simulink model "ODWRobot_KinematicModel"  (R2019b)
settings: Solver=ode5  StartTime=0.0  StopTime=10  FixedStep=Ts  RelTol=1e-3
undefined symbols (not defined in the file or in its folder): b, k1, k2, phi_init, rw, x_init, y_init
libraries: simulink x1
settings Model: Creator=kerrm  LastModifiedBy=kerrm
settings DataIOCC: ReturnWorkspaceOutputs=off

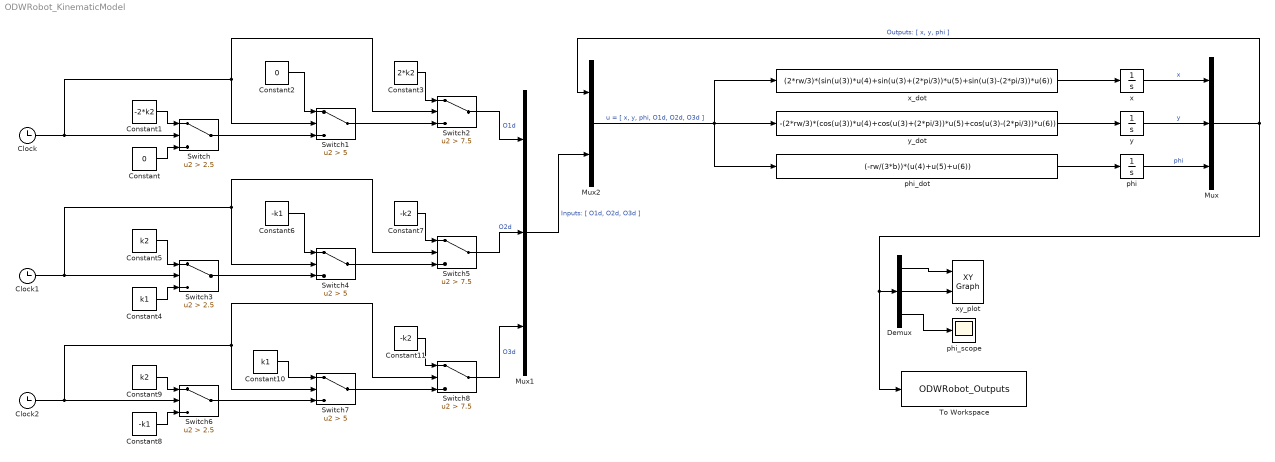
== system ODWRobot_KinematicModel ==
  Clock : Clock
  Clock1 : Clock
  Clock2 : Clock
  Constant : Constant  Value=0
  Constant1 : Constant  Value=-2*k2
  Constant10 : Constant  Value=k1
  Constant11 : Constant  Value=-k2
  Constant2 : Constant  Value=0
  Constant3 : Constant  Value=2*k2
  Constant4 : Constant  Value=k1
  Constant5 : Constant  Value=k2
  Constant6 : Constant  Value=-k1
  Constant7 : Constant  Value=-k2
  Constant8 : Constant  Value=-k1
  Constant9 : Constant  Value=k2
  Demux : Demux  Outputs=3
  Mux : Mux  Inputs=3
  Mux1 : Mux  Inputs=3
  Mux2 : Mux  Inputs=2
  Switch : Switch  Criteria=u2 > Threshold  Threshold=2.5
  Switch1 : Switch  Criteria=u2 > Threshold  Threshold=5
  Switch2 : Switch  Criteria=u2 > Threshold  Threshold=7.5
  Switch3 : Switch  Criteria=u2 > Threshold  Threshold=2.5
  Switch4 : Switch  Criteria=u2 > Threshold  Threshold=5
  Switch5 : Switch  Criteria=u2 > Threshold  Threshold=7.5
  Switch6 : Switch  Criteria=u2 > Threshold  Threshold=2.5
  Switch7 : Switch  Criteria=u2 > Threshold  Threshold=5
  Switch8 : Switch  Criteria=u2 > Threshold  Threshold=7.5
  To Workspace : ToWorkspace  VariableName=ODWRobot_Outputs  SampleTime=-1
      settings: Save2DSignal=2-D array (concatenate along first dimension)
  phi : Integrator  InitialCondition=phi_init
  phi_dot : Fcn  Expr=(-rw/(3*b))*(u(4)+u(5)+u(6))
  phi_scope : Scope
  x : Integrator  InitialCondition=x_init
  x_dot : Fcn  Expr=(2*rw/3)*(sin(u(3))*u(4)+sin(u(3)+(2*pi/3))*u(5)+sin(u(3)-(2*pi/3))*u(6))
  xy_plot : simulink/Sinks/XY Graph  xmin=-.1  xmax=1.1  ymin=-.1  ymax=1.1  st=-1
  y : Integrator  InitialCondition=y_init
  y_dot : Fcn  Expr=-(2*rw/3)*(cos(u(3))*u(4)+cos(u(3)+(2*pi/3))*u(5)+cos(u(3)-(2*pi/3))*u(6))
  wires:
  y/1 -> Mux/2  "y"
  phi/1 -> Mux/3  "phi"
  x/1 -> Mux/1  "x"
  Mux/1 -> To Workspace/1, Demux/1, Mux2/1  "Outputs: [ x, y, phi ]"
  Mux1/1 -> Mux2/2  "Inputs: [ O1d, O2d, O3d ]"
  Mux2/1 -> x_dot/1, phi_dot/1, y_dot/1  "u = [ x, y, phi, O1d, O2d, O3d ]"
  x_dot/1 -> x/1
  y_dot/1 -> y/1
  phi_dot/1 -> phi/1
  Demux/1 -> xy_plot/1
  Demux/2 -> xy_plot/2
  Demux/3 -> phi_scope/1
  Constant1/1 -> Switch/1
  Clock/1 -> Switch2/2, Switch1/2, Switch/2
  Constant/1 -> Switch/3
  Constant2/1 -> Switch1/1
  Switch/1 -> Switch1/3
  Switch1/1 -> Switch2/3
  Constant3/1 -> Switch2/1
  Switch2/1 -> Mux1/1  "O1d"
  Constant6/1 -> Switch4/1
  Constant4/1 -> Switch3/3
  Constant7/1 -> Switch5/1
  Constant5/1 -> Switch3/1
  Clock1/1 -> Switch4/2, Switch5/2, Switch3/2
  Switch3/1 -> Switch4/3
  Switch4/1 -> Switch5/3
  Switch7/1 -> Switch8/3
  Clock2/1 -> Switch8/2, Switch7/2, Switch6/2
  Switch6/1 -> Switch7/3
  Constant9/1 -> Switch6/1
  Constant10/1 -> Switch7/1
  Constant11/1 -> Switch8/1
  Constant8/1 -> Switch6/3
  Switch8/1 -> Mux1/3  "O3d"
  Switch5/1 -> Mux1/2  "O2d"
